simulink model "US53253_SimpleTorqueLimitingandGovernorControl"  (R2018b)
settings: Solver=ode45  StartTime=0.0  StopTime=10.0  RelTol=1e-3
undefined symbols (not defined in the file): DerivativeFilterGain_Gov, DerivativeFilterGain_Max, DerivativeFilterGain_Min, DerivativeFilterTimeConstant_Gov, DerivativeFilterTimeConstant_Max, DerivativeFilterTimeConstant_Min, DerivativeGainGovTable, DerivativeGainGovTable_X, DerivativeGainMaxTable, DerivativeGainMaxTable_X, DerivativeGainMinTable, DerivativeGainMinTable_X, DroopGovTable, DroopGovTable_X, DroopMaxTable, DroopMaxTable_X, DroopMinTable, DroopMinTable_X, FIZIT_GovSpeed, FIZIT_MaxSpeed, FIZIT_MinSpeed, FullThrottleSpeed_Gov, FullThrottleSpeed_Max, FullThrottleSpeed_Min, gov_maxspd, gov_minspd, GovTypeDefault, higpwr_C, higpwr_X, IntegralGainGovTable, IntegralGainGovTable_X, IntegralGainMinTable, IntegralGainMinTable_X, LIZIT_GovSpeed, LIZIT_MaxSpeed, LIZIT_MinSpeed, LowCoolantTempHysteresis, LowCoolantTempThreshold, lowpwr_C, lowpwr_X, LowSCRInletTempHysteresis, LowSCRInletTempThreshold, MinMaxTransitionHysteresis, nomfric_C, nomfric_X, nomfric_Y, NumberOfCylinders, ProportionalGainGovTable, ProportionalGainGovTable_X, ProportionalGainMaxTable, ProportionalGainMaxTable_X, ProportionalGainMinTable, ProportionalGainMinTable_X, SmkOp1_C, SmkOp1_X, SmkOp1_Y, ThrTqTbl_C, ThrTqTbl_X, ThrTqTbl_Y, TorqueToFuelConversionFactorInRangeTable_X ... (+8)
libraries: simulink x3, Filters x2
(part 1 of 2)
settings Model: Creator=ed50214  LastModifiedBy=dnyaneshwat2
settings DataIOCC: LimitDataPoints=on  SaveFormat=Array
settings OptimizationCC: BlockReduction=off  BooleanDataType=off  LifeSpan=inf
settings DebuggingCC: SaveWithParameterizedLinksMsg=none  UnderspecifiedInitializationDetection=Classic  MergeDetectMultiDrivingBlocksExec=none  SignalResolutionControl=TryResolveAllWithWarning  SFUnexpectedBacktrackingDiag=warning  SFNoUnconditionalDefaultTransitionDiag=warning  SFExecutionAtInitializationDiag=none
settings HardwareCC: ProdBitPerPointer=32  ProdBitPerSizeT=32  ProdBitPerPtrDiffT=32  ProdLargestAtomicFloat=None  ProdIntDivRoundTo=Undefined  ProdEndianess=Unspecified  ProdWordSize=32  ProdHWDeviceType=32-bit Generic  TargetUnknown=on
settings ModelReferenceCC: PropagateSignalLabelsOutOfModel=off
settings SFSimCC: SimUseLocalCustomCode=off
settings RTWCC: RTWUseLocalCustomCode=off
settings CodeAppCC: StateflowObjectComments=on
settings GRTTargetCC: TargetLangStandard=C89/C90 (ANSI)  GeneratePreprocessorConditionals=Disable all
settings ConfigComp: CovEnable=on  CovScope=ReferencedModels  RecordCoverage=on  CovMetricSettings=dw  CovHtmlReporting=on  CovSaveCumulativeToWorkspaceVar=on  CovSaveSingleToWorkspaceVar=on  CovExternalEMLEnable=off  CovSFcnEnable=off

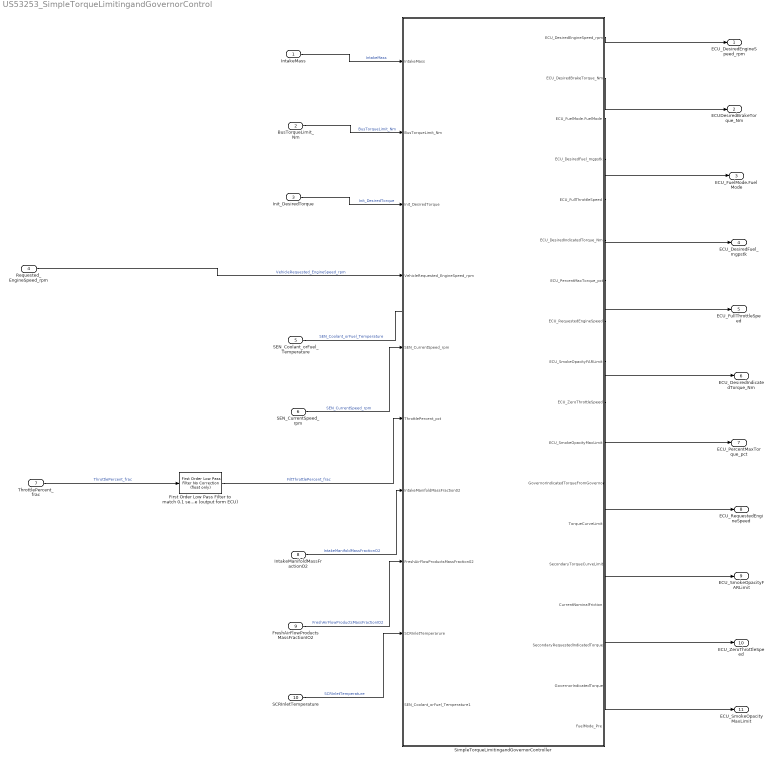
== system US53253_SimpleTorqueLimitingandGovernorControl ==
  IntakeMass : Inport
  BusTorqueLimit_Nm : Inport  Port=2
  Init_DesiredTorque : Inport  Port=3
  Requested_EngineSpeed_rpm : Inport  Port=4
  SEN_Coolant_orFuel_Temperature : Inport  Port=5
  SEN_CurrentSpeed_rpm : Inport  Port=6
  ThrottlePercent_frac : Inport  Port=7
  IntakeManifoldMassFractionO2 : Inport  Port=8
  FreshAirFlowProductsMassFractionIO2 : Inport  Port=9
  SCRInletTemperature : Inport  Port=10
  First Order Low Pass Filter to match 0.1 sec time constant in SiL from ThrottlePercent (input to ECU) to Throttle (output form ECU) : Filters/First Order Low Pass Filter No Correction (float only)  FilterGain=0.951229424500714  Filter_IC=0
      settings: SourceProductName=JDPS Filters
  SimpleTorqueLimitingandGovernorController : Subsystem  TreatAsAtomicUnit=on  mask(Engine control model){}
  ECU_DesiredEngineSpeed_rpm : Outport
  ECUDesiredBrakeTorque_Nm : Outport  Port=2
  ECU_FuelMode.FuelMode : Outport  Port=3
  ECU_DesiredFuel_mgpstk : Outport  Port=4
  ECU_FullThrottleSpeed : Outport  Port=5
  ECU_DesiredIndicatedTorque_Nm : Outport  Port=6
  ECU_PercentMaxTorque_pct : Outport  Port=7
  ECU_RequestedEngineSpeed : Outport  Port=8
  ECU_SmokeOpacityFARLimit : Outport  Port=9
  ECU_ZeroThrottleSpeed : Outport  Port=10
  ECU_SmokeOpacityMaxLimit : Outport  Port=11
  wires:
  IntakeMass/1 -> SimpleTorqueLimitingandGovernorController/1(IntakeMass)  "IntakeMass"
  BusTorqueLimit_Nm/1 -> SimpleTorqueLimitingandGovernorController/2(BusTorqueLimit_Nm)  "BusTorqueLimit_Nm"
  Init_DesiredTorque/1 -> SimpleTorqueLimitingandGovernorController/3(Init_DesiredTorque)  "Init_DesiredTorque"
  Requested_EngineSpeed_rpm/1 -> SimpleTorqueLimitingandGovernorController/4(VehicleRequested_EngineSpeed_rpm)  "VehicleRequested_EngineSpeed_rpm"
  SEN_Coolant_orFuel_Temperature/1 -> ?  "SEN_Coolant_orFuel_Temperature"
  SEN_CurrentSpeed_rpm/1 -> SimpleTorqueLimitingandGovernorController/5(SEN_CurrentSpeed_rpm)  "SEN_CurrentSpeed_rpm"
  IntakeManifoldMassFractionO2/1 -> SimpleTorqueLimitingandGovernorController/7(IntakeManifoldMassFraction02)  "IntakeManifoldMassFractionO2"
  FreshAirFlowProductsMassFractionIO2/1 -> SimpleTorqueLimitingandGovernorController/8(FreshAirFlowProductsMassFraction02)  "FreshAirFlowProductsMassFractionIO2"
  SCRInletTemperature/1 -> SimpleTorqueLimitingandGovernorController/9(SCRInletTemperarure)  "SCRInletTemperature"
  SimpleTorqueLimitingandGovernorController/1(ECU_DesiredEngineSpeed_rpm) -> ECU_DesiredEngineSpeed_rpm/1
  SimpleTorqueLimitingandGovernorController/2(ECU_DesiredBrakeTorque_Nm) -> ECUDesiredBrakeTorque_Nm/1
  SimpleTorqueLimitingandGovernorController/3(ECU_FuelMode.FuelMode) -> ECU_FuelMode.FuelMode/1
  SimpleTorqueLimitingandGovernorController/4(ECU_DesiredFuel_mgpstk) -> ECU_DesiredFuel_mgpstk/1
  SimpleTorqueLimitingandGovernorController/5(ECU_FullThrottleSpeed) -> ECU_FullThrottleSpeed/1
  SimpleTorqueLimitingandGovernorController/6(ECU_DesiredIndicatedTorque_Nm) -> ECU_DesiredIndicatedTorque_Nm/1
  SimpleTorqueLimitingandGovernorController/7(ECU_PercentMaxTorque_pct) -> ECU_PercentMaxTorque_pct/1
  SimpleTorqueLimitingandGovernorController/8(ECU_RequestedEngineSpeed) -> ECU_RequestedEngineSpeed/1
  SimpleTorqueLimitingandGovernorController/9(ECU_SmokeOpacityFARLimit) -> ECU_SmokeOpacityFARLimit/1
  SimpleTorqueLimitingandGovernorController/10(ECU_ZeroThrottleSpeed) -> ECU_ZeroThrottleSpeed/1
  SimpleTorqueLimitingandGovernorController/11(ECU_SmokeOpacityMaxLimit) -> ECU_SmokeOpacityMaxLimit/1
  ThrottlePercent_frac/1 -> First Order Low Pass Filter to match 0.1 sec time constant in SiL from ThrottlePercent (input to ECU) to Throttle (output form ECU)/1  "ThrottlePercent_frac"
  First Order Low Pass Filter to match 0.1 sec time constant in SiL from ThrottlePercent (input to ECU) to Throttle (output form ECU)/1 -> SimpleTorqueLimitingandGovernorController/6(ThrottlePercent_pct)  "FiltThrottlePercent_frac"

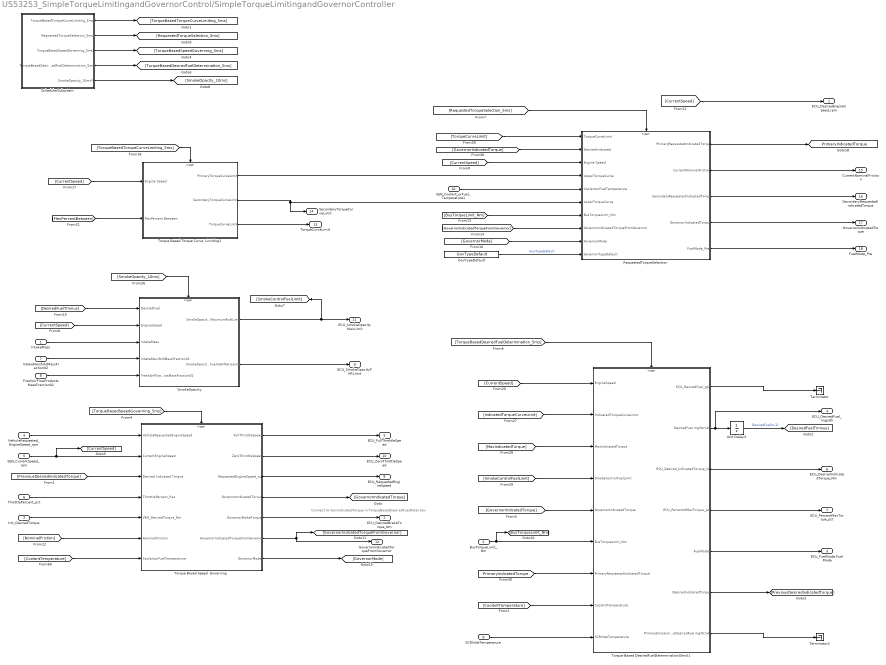
== system US53253_SimpleTorqueLimitingandGovernorControl/SimpleTorqueLimitingandGovernorController ==
  note: Connect to GovIndicatedTorque in TorqueBasedDesiredFuelDeter box
  IntakeMass : Inport
  BusTorqueLimit_Nm : Inport  Port=2
  Init_DesiredTorque : Inport  Port=3
  VehicleRequested_EngineSpeed_rpm : Inport  Port=4
  SEN_CurrentSpeed_rpm : Inport  Port=5
  ThrottlePercent_pct : Inport  Port=6
  IntakeManifoldMassFraction02 : Inport  Port=7
  FreshAirFlowProductsMassFraction02 : Inport  Port=8
  SCRInletTemperarure : Inport  Port=9
  SEN_Coolant_orFuel_Temperature1 : Inport  Port=10
  " Torque Based Speed  Governing" : Subsystem
  GovTypeDefault : Constant  Value=GovTypeDefault
  RequestedTorqueSelection : Subsystem
  SchedulerSubsytem : Stateflow chart  TreatAsAtomicUnit=on
  SmokeOpacity : Subsystem
  Terminator : Terminator
  Terminator2 : Terminator
  Torque Based DesiredFuelDetermination(5ms)1 : Subsystem
  Torque Based Torque Curve  Limiting1 : Subsystem
  Unit Delay3 : UnitDelay  InitialCondition=1000  SampleTime=-1
  ECU_DesiredEngineSpeed_rpm : Outport
  ECU_DesiredBrakeTorque_Nm : Outport  Port=2
  ECU_FuelMode.FuelMode : Outport  Port=3
  ECU_DesiredFuel_mgpstk : Outport  Port=4
  ECU_FullThrottleSpeed : Outport  Port=5
  ECU_DesiredIndicatedTorque_Nm : Outport  Port=6
  ECU_PercentMaxTorque_pct : Outport  Port=7
  ECU_RequestedEngineSpeed : Outport  Port=8
  ECU_SmokeOpacityFARLimit : Outport  Port=9
  ECU_ZeroThrottleSpeed : Outport  Port=10
  ECU_SmokeOpacityMaxLimit : Outport  Port=11
  GovernorIndicatedTorqueFromGovernor : Outport  Port=12
  TorqueCurveLimit : Outport  Port=13
  SecondaryTorqueCurveLimit : Outport  Port=14
  CurrentNominalFriction : Outport  Port=15
  SecondaryRequestedIndicatedTorque : Outport  Port=16
  GovernorIndicatedTorque : Outport  Port=17
  FuelMode_Pre : Outport  Port=18
  tag scope: PrimaryIndicatedTorque=global
  wires:
  [CurrentSpeed] -> ECU_DesiredEngineSpeed_rpm/1
  [SmokeOpacity_10ms] -> SmokeOpacity/Trigger
  [CurrentSpeed] -> SmokeOpacity/2(EngineSpeed)
  Unit Delay3/1 -> [DesiredFuelTminus]  "DesiredFuel(n-1)"
  [DesiredFuelTminus] -> SmokeOpacity/1(DesiredFuel)
  SmokeOpacity/2(SmokeOpacityFueltoAirRatioLimit) -> ECU_SmokeOpacityFARLimit/1
  Torque Based DesiredFuelDetermination(5ms)1/5(FuelMode) -> ECU_FuelMode.FuelMode/1
  Torque Based DesiredFuelDetermination(5ms)1/2(DesiredFuel mg/Stroke) -> ECU_DesiredFuel_mgpstk/1, Unit Delay3/1
  VehicleRequested_EngineSpeed_rpm/1 -> " Torque Based Speed  Governing"/1(VehicleRequestedEngineSpeed)
  SEN_CurrentSpeed_rpm/1 -> [CurrentSpeed], " Torque Based Speed  Governing"/2(CurrentEngineSpeed)
  Torque Based DesiredFuelDetermination(5ms)1/3(ECU_Desired_IndicatedTorque_Nm) -> ECU_DesiredIndicatedTorque_Nm/1
  Torque Based DesiredFuelDetermination(5ms)1/4(ECU_PercentofMaxTorque_pct) -> ECU_PercentMaxTorque_pct/1
  Torque Based DesiredFuelDetermination(5ms)1/7(PrimaryEmissionsMapDesiredFuel mg/Stroke) -> Terminator2/1
  [PreviousDesiredIndicatedTorque] -> " Torque Based Speed  Governing"/3(Desired Indicated Torque)
  " Torque Based Speed  Governing"/4(GovernorIndicatedTorque) -> [GovernorIndicatedTorque]
  [GovernorIndicatedTorque] -> Torque Based DesiredFuelDetermination(5ms)1/5(GovernorIndicatedTorque)
  Torque Based DesiredFuelDetermination(5ms)1/1(ECU_DesiredFuel_gps) -> Terminator/1
  [NominalFriction] -> " Torque Based Speed  Governing"/6(NominalFriction)
  Init_DesiredTorque/1 -> " Torque Based Speed  Governing"/5(VEH_DesiredTorque_Nm)
  BusTorqueLimit_Nm/1 -> [BusTorqueLimit_Nm], Torque Based DesiredFuelDetermination(5ms)1/6(BusTorqueLimit_Nm)
  IntakeMass/1 -> SmokeOpacity/3(IntakeMass)
  ThrottlePercent_pct/1 -> " Torque Based Speed  Governing"/4(ThrottlePercent_frac)
  " Torque Based Speed  Governing"/1(FullThrottleSpeed) -> ECU_FullThrottleSpeed/1
  " Torque Based Speed  Governing"/2(ZeroThrottleSpeed) -> ECU_ZeroThrottleSpeed/1
  " Torque Based Speed  Governing"/3(RequestedEngineSpeed_out) -> ECU_RequestedEngineSpeed/1
  [CurrentSpeed] -> Torque Based DesiredFuelDetermination(5ms)1/1(EngineSpeed)
  [PrimaryIndicatedTorque] -> Torque Based DesiredFuelDetermination(5ms)1/7(PrimaryRequestedIndicatedTorque)
  Torque Based DesiredFuelDetermination(5ms)1/6(DesiredIndicatedTorque) -> [PreviousDesiredIndicatedTorque]
  [IndicatedTorqueCurveLimit] -> Torque Based DesiredFuelDetermination(5ms)1/2(IndicatedTorqueCurveLimit)
  [SmokeControlFuelLimit] -> Torque Based DesiredFuelDetermination(5ms)1/4(SmokeControlFuelLimit)
  [MaxIndicatedTorque] -> Torque Based DesiredFuelDetermination(5ms)1/3(MaxIndicatedTorque)
  SmokeOpacity/1(SmokeOpacityMaximumFuelLimit) -> ECU_SmokeOpacityMaxLimit/1, [SmokeControlFuelLimit]
  [GovernorIndicatedTorque] -> RequestedTorqueSelection/2(DesiredInidcated)
  RequestedTorqueSelection/1(PrimaryRequestedIndicatedTorque) -> [PrimaryIndicatedTorque]
  [TorqueCurveLimit] -> RequestedTorqueSelection/1(TorqueCurveLimit)
  [CoolantTemperature] -> " Torque Based Speed  Governing"/7(CoolantorFuelTemperature)
  FreshAirFlowProductsMassFraction02/1 -> SmokeOpacity/5(FreshAirFlowProductsMassFraction02)
  IntakeManifoldMassFraction02/1 -> SmokeOpacity/4(IntakeManifoldMassFraction02)
  " Torque Based Speed  Governing"/5(GovernorBrakeTorque) -> ECU_DesiredBrakeTorque_Nm/1
  [CoolantTemperature] -> Torque Based DesiredFuelDetermination(5ms)1/8(CoolantTemperature)
  SCRInletTemperarure/1 -> Torque Based DesiredFuelDetermination(5ms)1/9(SCRInletTemperature)
  [TorqueBasedSpeedGoverning_5ms] -> " Torque Based Speed  Governing"/Trigger
  [TorqueBasedDesiredFuelDetermination_5ms] -> Torque Based DesiredFuelDetermination(5ms)1/Trigger
  [RequestedTorqueSelection_5ms] -> RequestedTorqueSelection/Trigger
  SchedulerSubsytem/1(TorqueBasedTorqueCurveLimiting_5ms()) -> [TorqueBasedTorqueCurveLimiting_5ms]
  SchedulerSubsytem/2(RequestedTorqueSelection_5ms()) -> [RequestedTorqueSelection_5ms]
  SchedulerSubsytem/3(TorqueBasedSpeedGoverning_5ms()) -> [TorqueBasedSpeedGoverning_5ms]
  SchedulerSubsytem/4(TorqueBasedDesiredFuelDetermination_5ms()) -> [TorqueBasedDesiredFuelDetermination_5ms]
  SchedulerSubsytem/5(SmokeOpacity_10ms()) -> [SmokeOpacity_10ms]
  [CurrentSpeed] -> RequestedTorqueSelection/3(Engine Speed)
  SEN_Coolant_orFuel_Temperature1/1 -> RequestedTorqueSelection/5(CoolantorFuelTemperature)
  [BusTorqueLimit_Nm] -> RequestedTorqueSelection/7(BusTorqueLimit_Nm)
  " Torque Based Speed  Governing"/6(GovernorIndicatedTorqueFromGovernor) -> GovernorIndicatedTorqueFromGovernor/1, [GovernorIndicatedTorqueFromGovernor]
  [GovernorIndicatedTorqueFromGovernor] -> RequestedTorqueSelection/8(GovernorIndicatedTorqueFromGovernor)
  [GovernorMode] -> RequestedTorqueSelection/9(GovernorMode)
  " Torque Based Speed  Governing"/7(GovernorMode) -> [GovernorMode]
  GovTypeDefault/1 -> RequestedTorqueSelection/10(GovernorTypeDefault)  "GovTypeDefault"
  Torque Based Torque Curve  Limiting1/2(SecondaryTorqueCurveLimit) -> RequestedTorqueSelection/6(LowerTorqueCurve), SecondaryTorqueCurveLimit/1
  Torque Based Torque Curve  Limiting1/3(TorqueCurveLimit) -> TorqueCurveLimit/1
  [TorqueBasedTorqueCurveLimiting_5ms] -> Torque Based Torque Curve  Limiting1/Trigger
  [FlexPercentBetween] -> Torque Based Torque Curve  Limiting1/2(FlexPercent Between)
  [CurrentSpeed] -> Torque Based Torque Curve  Limiting1/1(Engine Speed)
  Torque Based Torque Curve  Limiting1/1(PrimaryTorqueCurveLimit) -> RequestedTorqueSelection/4(UpperTorqueCurve)
  RequestedTorqueSelection/2(CurrentNominalFriction) -> CurrentNominalFriction/1
  RequestedTorqueSelection/3(SecondaryRequestedIndicatedTorque) -> SecondaryRequestedIndicatedTorque/1
  RequestedTorqueSelection/4(GovernorIndicatedTorque) -> GovernorIndicatedTorque/1
  RequestedTorqueSelection/5(FuelMode_Pre) -> FuelMode_Pre/1

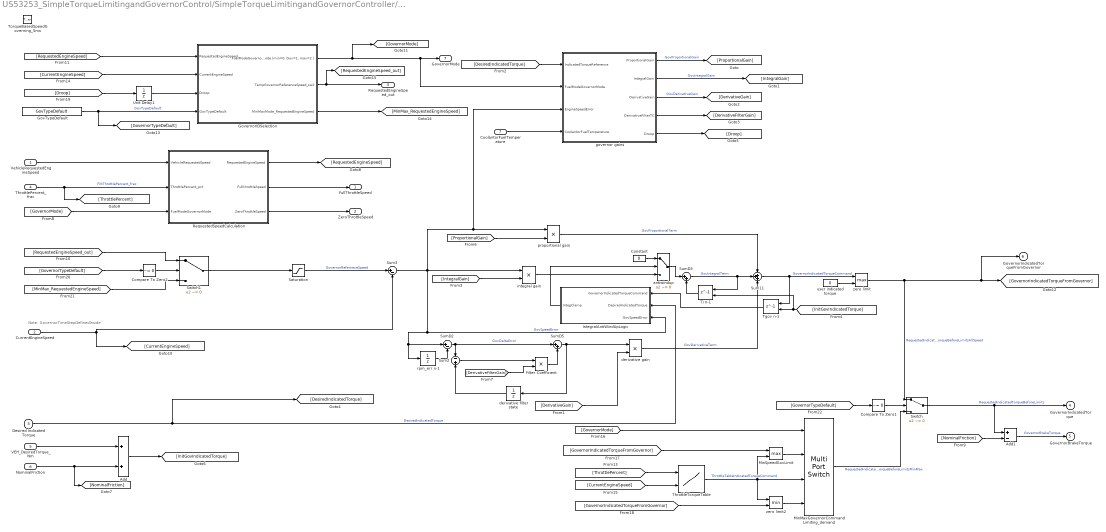
== system US53253_SimpleTorqueLimitingandGovernorControl/SimpleTorqueLimitingandGovernorController/ Torque Based Speed  Governing ==
  note: Note: GovernorTimeStepDefinedInside
  VehicleRequestedEngineSpeed : Inport
  CurrentEngineSpeed : Inport  Port=2
  Desired Indicated Torque : Inport  Port=3
  ThrottlePercent_frac : Inport  Port=4
  VEH_DesiredTorque_Nm : Inport  Port=5
  NominalFriction : Inport  Port=6
  CoolantorFuelTemperature : Inport  Port=7
  TorqueBasedSpeedGoverning_5ms : TriggerPort  TriggerType=function-call  VariantControl=(inherit)  PortDimensions=1
  Add : Sum
  Add1 : Sum  Inputs=+-
  Compare To Zero1 : simulink/Logic and Bit Operations/Compare To Zero  relop=~=  OutDataTypeStr=uint8
  Compare To Zero2 : simulink/Logic and Bit Operations/Compare To Zero  relop=~=  OutDataTypeStr=uint8
  Constant : Constant  Value=0
  Filter Coefficient : Product  Inputs=**  RndMeth=Zero
  GovTypeDefault : Constant  Value=GovTypeDefault
  GovernorIDSelection : Subsystem
  IntegralAntiWindUpLogic : Stateflow chart  TreatAsAtomicUnit=on
  MinMaxGovernorCommandLimiting_demand : MultiPortSwitch  DataPortOrder=Zero-based contiguous  zeroidx=on
  MinSpeedGovLimit : MinMax  Function=max  Inputs=2
  RequestedSpeedCalculation : Subsystem
  Saturation : Saturate  UpperLimit=gov_maxspd  LowerLimit=gov_minspd
      settings: AttributesFormatString=<lim: %<LowerLimit>/%<UpperLimit>>
  Sum11 : Sum  DisableCoverage=on  Inputs=+++
  Sum2 : Sum  Inputs=-+
  Sum3 : Sum  Inputs=|+-
  SumD2 : Sum  DisableCoverage=on  Inputs=|+-
  SumD3 : Sum  DisableCoverage=on  Inputs=|++
  SumD5 : Sum  DisableCoverage=on  Inputs=|++
  Switch : Switch  Criteria=u2 ~= 0
  Switch1 : Switch  Criteria=u2 ~= 0
  Tgov n-1 : Delay  DelayLength=1  InitialConditionSource=Input port
      settings: InputPortMap=u0,p4
  ThrottleTorqueTable : Lookup_n-D  BreakpointsForDimension1=ThrTqTbl_X  BreakpointsForDimension2=ThrTqTbl_Y  Table=ThrTqTbl_C  ExtrapMethod=Clip  UseLastTableValue=on  RndMeth=Simplest  InputSameDT=on
  Ti n-1 : Delay  DelayLength=1  InitialConditionSource=Input port
      settings: InputPortMap=u0,p4
  Unit Delay1 : UnitDelay  SampleTime=-1
  antiwindup : Switch  Criteria=u2 ~= 0
  derivative filter state : UnitDelay  SampleTime=-1
  derivative gain : Product  RndMeth=Zero
  governor gains : Subsystem
  integral gain : Product  RndMeth=Zero
  proportional gain : Product  RndMeth=Zero
  rpm_err n-1 : UnitDelay  SampleTime=-1
  user indicated torque : Constant  Value=0
  zero limit : MinMax  Function=max  Inputs=2
  zero limit2 : MinMax  Inputs=2
  FullThrottleSpeed : Outport
  ZeroThrottleSpeed : Outport  Port=2
  RequestedEngineSpeed_out : Outport  Port=3
  GovernorIndicatedTorque : Outport  Port=4  InitialOutput=0
  GovernorBrakeTorque : Outport  Port=5  InitialOutput=0
  GovernorIndicatedTorqueFromGovernor : Outport  Port=6  InitialOutput=0
  GovernorMode : Outport  Port=7
  wires:
  Desired Indicated Torque/1 -> [DesiredIndicatedTorque], IntegralAntiWindUpLogic/2(DesiredIndicatedTorque)  "DesiredIndicatedTorque"
  Tgov n-1/1 -> IntegralAntiWindUpLogic/1(GovernorIndicatedTorqueCommand)
  Ti n-1/1 -> SumD3/2
  Sum3/1 -> IntegralAntiWindUpLogic/3(GovSpeedError), SumD2/1, rpm_err n-1/1, integral gain/1, proportional gain/1, governor gains/3(EngineSpeedError)  "GovSpeedError"
  SumD3/1 -> Sum11/2, Ti n-1/1  "GovIntegralTerm"
  proportional gain/1 -> Sum11/1  "GovProportionalTerm"
  Sum11/1 -> zero limit/1, Tgov n-1/1  "GovernorIndicatedTorqueCommand"
  antiwindup/1 -> SumD3/1
  integral gain/1 -> antiwindup/3
  derivative gain/1 -> Sum11/3  "GovDerivativeTerm"
  Constant/1 -> antiwindup/1
  [ProportionalGain] -> proportional gain/2
  [IntegralGain] -> integral gain/2
  governor gains/1(ProportionalGain) -> [ProportionalGain]  "GovProportionalGain"
  CurrentEngineSpeed/1 -> [CurrentEngineSpeed], Sum3/2
  user indicated torque/1 -> zero limit/2
  [DerivativeGain] -> derivative gain/2
  governor gains/2(IntegralGain) -> [IntegralGain]  "GovIntegralGain"
  [DesiredIndicatedTorque] -> governor gains/1(IndicatedTorqueReference)
  governor gains/5(Droop) -> [Droop]
  governor gains/4(DerivativeFilterTC) -> [DerivativeFilterGain]
  governor gains/3(DerivativeGain) -> [DerivativeGain]  "GovDerivativeGain"
  SumD5/1 -> derivative filter state/1, derivative gain/1
  Sum2/1 -> Filter Coefficient/1
  [DerivativeFilterGain] -> Filter Coefficient/2
  SumD2/1 -> SumD5/1, Sum2/1  "GovDeltaError"
  rpm_err n-1/1 -> SumD2/2
  Saturation/1 -> Sum3/1  "GovernorReferneceSpeed"
  [InitGovIndicatedTorque] -> Tgov n-1/2, Ti n-1/2
  VehicleRequestedEngineSpeed/1 -> RequestedSpeedCalculation/1(VehicleRequestedSpeed)
  ThrottlePercent_frac/1 -> [ThrottlePercent], RequestedSpeedCalculation/2(ThrottlePercent_pct)  "FiltThrottlePercent_frac"
  [GovernorMode] -> RequestedSpeedCalculation/3(FuelModeGovernorMode)
  RequestedSpeedCalculation/1(RequestedEngineSpeed) -> [RequestedEngineSpeed]
  [RequestedEngineSpeed] -> GovernorIDSelection/1(RequestedEngineSpeed)
  RequestedSpeedCalculation/3(ZeroThrottleSpeed) -> ZeroThrottleSpeed/1
  RequestedSpeedCalculation/2(FullthrottleSpeed) -> FullThrottleSpeed/1
  CoolantorFuelTemperature/1 -> governor gains/4(CoolantorFuelTemperature)
  Compare To Zero1/1 -> Switch/2
  [ThrottlePercent] -> ThrottleTorqueTable/1
  [CurrentEngineSpeed] -> ThrottleTorqueTable/2
  [GovernorMode] -> MinMaxGovernorCommandLimiting_demand/1
  MinMaxGovernorCommandLimiting_demand/1 -> Switch/3  "RequestedIndicatedTorqueBeforeLimitsMinMax"
  ThrottleTorqueTable/1 -> MinSpeedGovLimit/2, zero limit2/1, MinMaxGovernorCommandLimiting_demand/3  "ThrottleTableIndicatedTorqueCommand"
  [GovernorIndicatedTorqueFromGovernor] -> MinSpeedGovLimit/1
  [GovernorIndicatedTorqueFromGovernor] -> zero limit2/2
  GovernorIDSelection/1("FuelModeGovernorMode (min=0, Gov=1, max=2 )") -> governor gains/2(FuelModeGovernorMode), GovernorMode/1, [GovernorMode]
  zero limit/1 -> GovernorIndicatedTorqueFromGovernor/1, [GovernorIndicatedTorqueFromGovernor], Switch/1  "RequestedIndicatedTorqueBeforeLimitsAllSpeed"
  Switch/1 -> Add1/1, GovernorIndicatedTorque/1  "RequestedIndicatedTorqueBeforeLimits"
  MinSpeedGovLimit/1 -> MinMaxGovernorCommandLimiting_demand/2
  zero limit2/1 -> MinMaxGovernorCommandLimiting_demand/4
  [CurrentEngineSpeed] -> GovernorIDSelection/2(CurrentEngineSpeed)
  [Droop] -> Unit Delay1/1
  Unit Delay1/1 -> GovernorIDSelection/3(Droop)
  GovernorIDSelection/3(MinMaxMode_RequestedEngineSpeed) -> [MinMax_RequestedEngineSpeed]
  [GovernorTypeDefault] -> Compare To Zero2/1
  Switch1/1 -> Saturation/1
  [RequestedEngineSpeed_out] -> Switch1/1
  Compare To Zero2/1 -> Switch1/2
  [MinMax_RequestedEngineSpeed] -> Switch1/3
  [GovernorTypeDefault] -> Compare To Zero1/1
  Add/1 -> [InitGovIndicatedTorque]
  VEH_DesiredTorque_Nm/1 -> Add/1
  NominalFriction/1 -> [NominalFriction], Add/2
  [NominalFriction] -> Add1/2
  Add1/1 -> GovernorBrakeTorque/1  "GovernorBrakeTorque"
  GovTypeDefault/1 -> [GovernorTypeDefault], GovernorIDSelection/4(GovTypeDefault)  "GovTypeDefault"
  Filter Coefficient/1 -> SumD5/2
  derivative filter state/1 -> Sum2/2
  GovernorIDSelection/2(TempGovernorReferenceSpeed_sw2) -> [RequestedEngineSpeed_out], RequestedEngineSpeed_out/1
  IntegralAntiWindUpLogic/1(IntegClamp) -> antiwindup/2

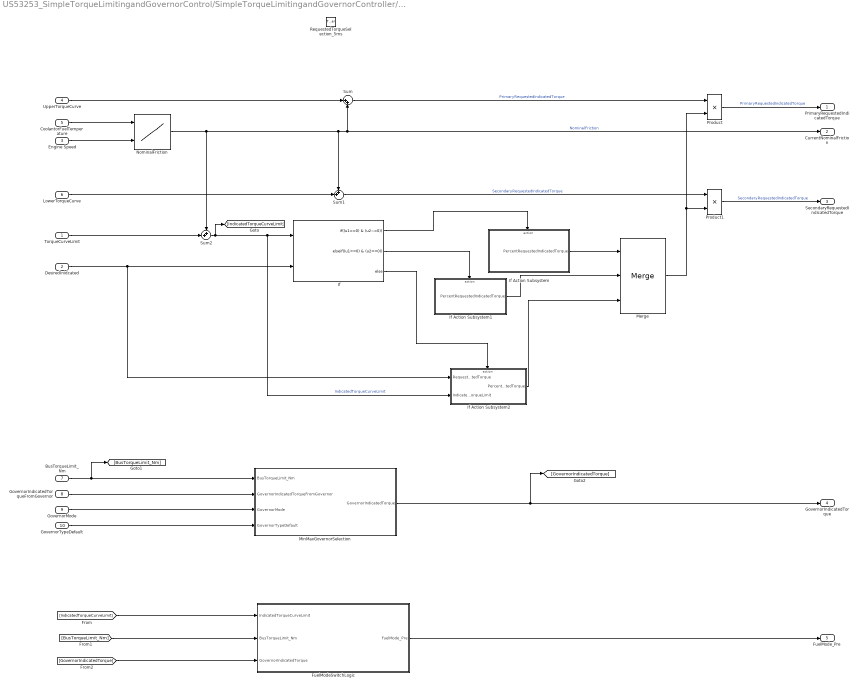
== system US53253_SimpleTorqueLimitingandGovernorControl/SimpleTorqueLimitingandGovernorController/RequestedTorqueSelection ==
  TorqueCurveLimit : Inport
  DesiredInidcated : Inport  Port=2
  Engine Speed : Inport  Port=3
  UpperTorqueCurve : Inport  Port=4
  CoolantorFuelTemperature : Inport  Port=5
  LowerTorqueCurve : Inport  Port=6
  BusTorqueLimit_Nm : Inport  Port=7
  GovernorIndicatedTorqueFromGovernor : Inport  Port=8
  GovernorMode : Inport  Port=9
  GovernorTypeDefault : Inport  Port=10
  RequestedTorqueSelection_5ms : TriggerPort  TriggerType=function-call  VariantControl=(inherit)  PortDimensions=1
  FuelModeSwitchLogic : Subsystem
  If : If  NumInputs=2  IfExpression=(u1==0) & (u2~=0)  ElseIfExpressions=(u1==0) & (u2==0)
  If Action Subsystem : Subsystem  TreatAsAtomicUnit=on
  If Action Subsystem1 : Subsystem  TreatAsAtomicUnit=on
  If Action Subsystem2 : Subsystem  TreatAsAtomicUnit=on
  Merge : Merge  Inputs=3
  MinMaxGovernorSelection : Subsystem
  NominalFriction : Lookup_n-D  BreakpointsForDimension1=nomfric_Y  BreakpointsForDimension2=nomfric_X  Table=nomfric_C  ExtrapMethod=Clip  UseLastTableValue=on  RndMeth=Simplest  InputSameDT=on
  Product : Product  RndMeth=Zero
  Product1 : Product  RndMeth=Zero
  Sum : Sum  Inputs=|++
  Sum1 : Sum  Inputs=++|
  Sum2 : Sum  Inputs=++|
  PrimaryRequestedIndicatedTorque : Outport
  CurrentNominalFriction : Outport  Port=2
  SecondaryRequestedIndicatedTorque : Outport  Port=3
  GovernorIndicatedTorque : Outport  Port=4
  FuelMode_Pre : Outport  Port=5
  wires:
  UpperTorqueCurve/1 -> Sum/1
  DesiredInidcated/1 -> If Action Subsystem2/1(RequestedIndicatedTorque), If/2
  TorqueCurveLimit/1 -> Sum2/2
  Sum/1 -> Product/1  "PrimaryRequestedIndicatedTorque"
  Product/1 -> PrimaryRequestedIndicatedTorque/1  "PrimaryRequestedIndicatedTorque"
  CoolantorFuelTemperature/1 -> NominalFriction/1
  Engine Speed/1 -> NominalFriction/2
  NominalFriction/1 -> CurrentNominalFriction/1, Sum/2, Sum1/1, Sum2/1  "NominalFriction"
  LowerTorqueCurve/1 -> Sum1/2
  If/1 -> If Action Subsystem/Action
  If Action Subsystem/1(PercentRequestedIndicatedTorque) -> Merge/1
  Product1/1 -> SecondaryRequestedIndicatedTorque/1  "SecondaryRequestedIndicatedTorque"
  Sum1/1 -> Product1/1  "SecondaryRequestedIndicatedTorque"
  If Action Subsystem1/1(PercentRequestedIndicatedTorque) -> Merge/2
  If Action Subsystem2/1(PercentRequestedIndicatedTorque) -> Merge/3
  If/3 -> If Action Subsystem2/Action
  If/2 -> If Action Subsystem1/Action
  Sum2/1 -> [IndicatedTorqueCurveLimit], If Action Subsystem2/2(IndicatedTorqueLimit), If/1  "IndicatedTorqueCurveLimit"
  Merge/1 -> Product/2, Product1/2
  [IndicatedTorqueCurveLimit] -> FuelModeSwitchLogic/1(IndicatedTorqueCurveLimit)
  [BusTorqueLimit_Nm] -> FuelModeSwitchLogic/2(BusTorqueLimit_Nm)
  [GovernorIndicatedTorque] -> FuelModeSwitchLogic/3(GovernorIndicatedTorque)
  FuelModeSwitchLogic/1(FuelMode_Pre) -> FuelMode_Pre/1
  BusTorqueLimit_Nm/1 -> [BusTorqueLimit_Nm], MinMaxGovernorSelection/1(BusTorqueLimit_Nm)
  GovernorIndicatedTorqueFromGovernor/1 -> MinMaxGovernorSelection/2(GovernorIndicatedTorqueFromGovernor)
  GovernorMode/1 -> MinMaxGovernorSelection/3(GovernorMode)
  GovernorTypeDefault/1 -> MinMaxGovernorSelection/4(GovernorTypeDefault)
  MinMaxGovernorSelection/1(GovernorIndicatedTorque) -> [GovernorIndicatedTorque], GovernorIndicatedTorque/1

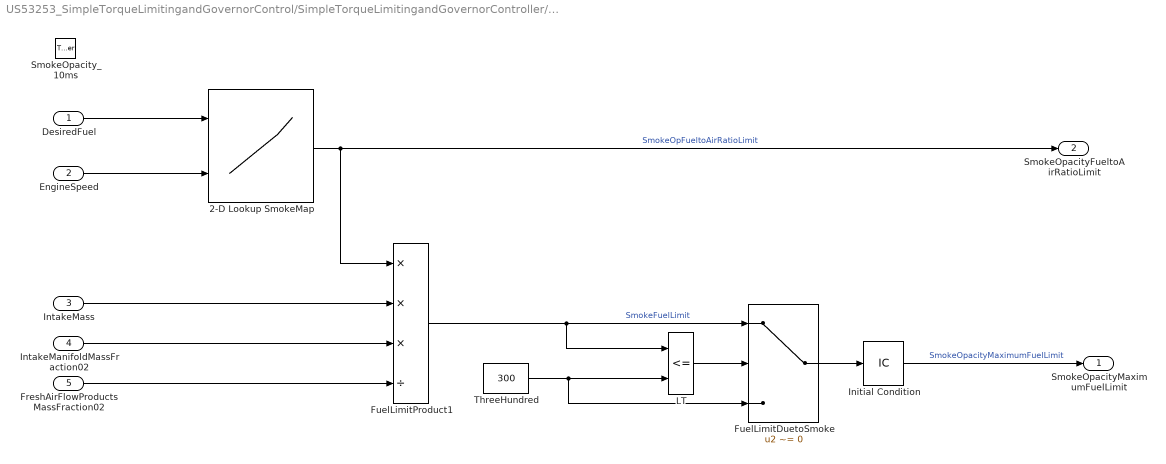
== system US53253_SimpleTorqueLimitingandGovernorControl/SimpleTorqueLimitingandGovernorController/SmokeOpacity ==
  DesiredFuel : Inport
  EngineSpeed : Inport  Port=2
  IntakeMass : Inport  Port=3
  IntakeManifoldMassFraction02 : Inport  Port=4
  FreshAirFlowProductsMassFraction02 : Inport  Port=5
  SmokeOpacity_10ms : TriggerPort  TriggerType=function-call  VariantControl=(inherit)  PortDimensions=1
  2-D Lookup SmokeMap : Lookup_n-D  BreakpointsForDimension1=SmkOp1_Y  BreakpointsForDimension2=SmkOp1_X  Table=SmkOp1_C  ExtrapMethod=Clip  UseLastTableValue=on  RndMeth=Simplest  InputSameDT=on
  FuelLimitDuetoSmoke : Switch  Criteria=u2 ~= 0
  FuelLimitProduct1 : Product  Inputs=***/  SaturateOnIntegerOverflow=on
  Initial Condition : InitialCondition  Value=500
  LT : RelationalOperator  Operator=<=  OutDataTypeStr=boolean  RndMeth=Nearest
  ThreeHundred : Constant  Value=300
  SmokeOpacityMaximumFuelLimit : Outport
  SmokeOpacityFueltoAirRatioLimit : Outport  Port=2
  wires:
  DesiredFuel/1 -> 2-D Lookup SmokeMap/1
  EngineSpeed/1 -> 2-D Lookup SmokeMap/2
  2-D Lookup SmokeMap/1 -> SmokeOpacityFueltoAirRatioLimit/1, FuelLimitProduct1/1  "SmokeOpFueltoAirRatioLimit"
  FuelLimitDuetoSmoke/1 -> Initial Condition/1
  LT/1 -> FuelLimitDuetoSmoke/2
  ThreeHundred/1 -> LT/2, FuelLimitDuetoSmoke/3
  FuelLimitProduct1/1 -> LT/1, FuelLimitDuetoSmoke/1  "SmokeFuelLimit"
  IntakeMass/1 -> FuelLimitProduct1/2
  IntakeManifoldMassFraction02/1 -> FuelLimitProduct1/3
  FreshAirFlowProductsMassFraction02/1 -> FuelLimitProduct1/4
  Initial Condition/1 -> SmokeOpacityMaximumFuelLimit/1  "SmokeOpacityMaximumFuelLimit"

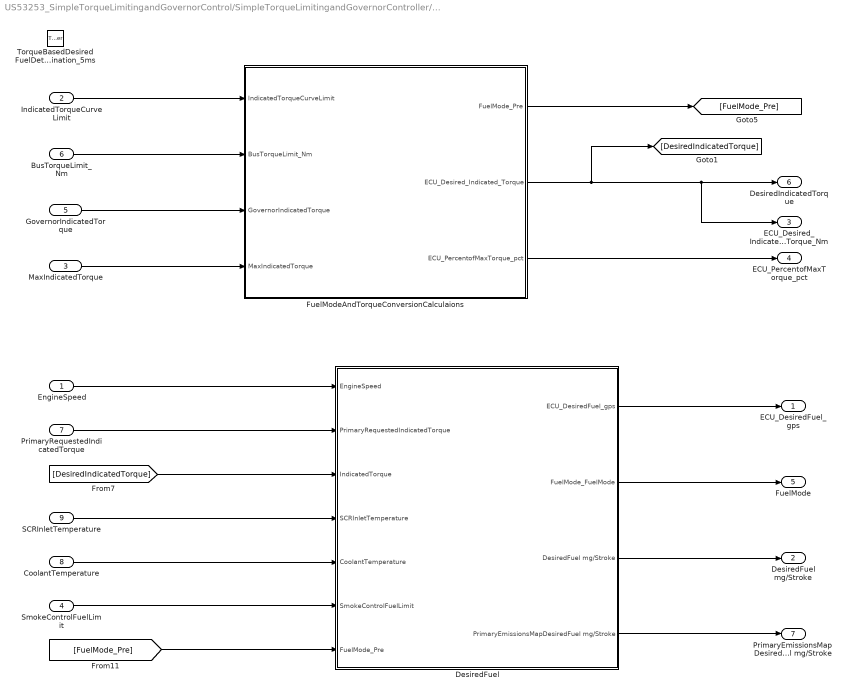
== system US53253_SimpleTorqueLimitingandGovernorControl/SimpleTorqueLimitingandGovernorController/Torque Based DesiredFuelDetermination(5ms)1 ==
  EngineSpeed : Inport
  IndicatedTorqueCurveLimit : Inport  Port=2
  MaxIndicatedTorque : Inport  Port=3
  SmokeControlFuelLimit : Inport  Port=4
  GovernorIndicatedTorque : Inport  Port=5
  BusTorqueLimit_Nm : Inport  Port=6
  PrimaryRequestedIndicatedTorque : Inport  Port=7
  CoolantTemperature : Inport  Port=8
  SCRInletTemperature : Inport  Port=9
  TorqueBasedDesiredFuelDetermination_5ms : TriggerPort  TriggerType=function-call  VariantControl=(inherit)  PortDimensions=1
  DesiredFuel : Subsystem
  FuelModeAndTorqueConversionCalculaions : Subsystem
  ECU_DesiredFuel_gps : Outport
  DesiredFuel mg/Stroke : Outport  Port=2
  ECU_Desired_IndicatedTorque_Nm : Outport  Port=3
  ECU_PercentofMaxTorque_pct : Outport  Port=4
  FuelMode : Outport  Port=5
  DesiredIndicatedTorque : Outport  Port=6
  PrimaryEmissionsMapDesiredFuel mg/Stroke : Outport  Port=7
  wires:
  EngineSpeed/1 -> DesiredFuel/1(EngineSpeed)
  [DesiredIndicatedTorque] -> DesiredFuel/3(IndicatedTorque)
  PrimaryRequestedIndicatedTorque/1 -> DesiredFuel/2(PrimaryRequestedIndicatedTorque)
  SCRInletTemperature/1 -> DesiredFuel/4(SCRInletTemperature)
  CoolantTemperature/1 -> DesiredFuel/5(CoolantTemperature)
  FuelModeAndTorqueConversionCalculaions/2(ECU_Desired_Indicated_Torque) -> [DesiredIndicatedTorque], ECU_Desired_IndicatedTorque_Nm/1, DesiredIndicatedTorque/1
  IndicatedTorqueCurveLimit/1 -> FuelModeAndTorqueConversionCalculaions/1(IndicatedTorqueCurveLimit)
  BusTorqueLimit_Nm/1 -> FuelModeAndTorqueConversionCalculaions/2(BusTorqueLimit_Nm)
  GovernorIndicatedTorque/1 -> FuelModeAndTorqueConversionCalculaions/3(GovernorIndicatedTorque)
  MaxIndicatedTorque/1 -> FuelModeAndTorqueConversionCalculaions/4(MaxIndicatedTorque)
  FuelModeAndTorqueConversionCalculaions/1(FuelMode_Pre) -> [FuelMode_Pre]
  FuelModeAndTorqueConversionCalculaions/3(ECU_PercentofMaxTorque_pct) -> ECU_PercentofMaxTorque_pct/1
  DesiredFuel/1(ECU_DesiredFuel_gps) -> ECU_DesiredFuel_gps/1
  DesiredFuel/2(FuelMode_FuelMode) -> FuelMode/1
  DesiredFuel/3(DesiredFuel mg/Stroke) -> DesiredFuel mg/Stroke/1
  DesiredFuel/4(PrimaryEmissionsMapDesiredFuel mg/Stroke) -> PrimaryEmissionsMapDesiredFuel mg/Stroke/1
  SmokeControlFuelLimit/1 -> DesiredFuel/6(SmokeControlFuelLimit)
  [FuelMode_Pre] -> DesiredFuel/7(FuelMode_Pre)

== system US53253_SimpleTorqueLimitingandGovernorControl/SimpleTorqueLimitingandGovernorController/Torque Based Torque Curve  Limiting1 ==
  Engine Speed : Inport
  FlexPercent Between : Inport  Port=2
  TorqueBasedTorqueCurveLimiting_5ms : TriggerPort  TriggerType=function-call  VariantControl=(inherit)  PortDimensions=1
  Lower Curve : Lookup  InputValues=lowpwr_X  Table=lowpwr_C  LookUpMeth=Interpolation-Use End Values
  Product : Product
  Sum1 : Sum  Inputs=|+-
  Sum2 : Sum  Inputs=|++
  Upper Curve : Lookup  InputValues=higpwr_X  Table=higpwr_C  LookUpMeth=Interpolation-Use End Values
  PrimaryTorqueCurveLimit : Outport
  SecondaryTorqueCurveLimit : Outport  Port=2
  TorqueCurveLimit : Outport  Port=3
  wires:
  Engine Speed/1 -> Upper Curve/1, Lower Curve/1
  Upper Curve/1 -> PrimaryTorqueCurveLimit/1, Sum1/1  "UpperTorqueCurve"
  Lower Curve/1 -> SecondaryTorqueCurveLimit/1, Sum2/2, Sum1/2  "LowerTorqueCurve"
  Sum1/1 -> Product/2
  FlexPercent Between/1 -> Product/1
  Product/1 -> Sum2/1
  Sum2/1 -> TorqueCurveLimit/1

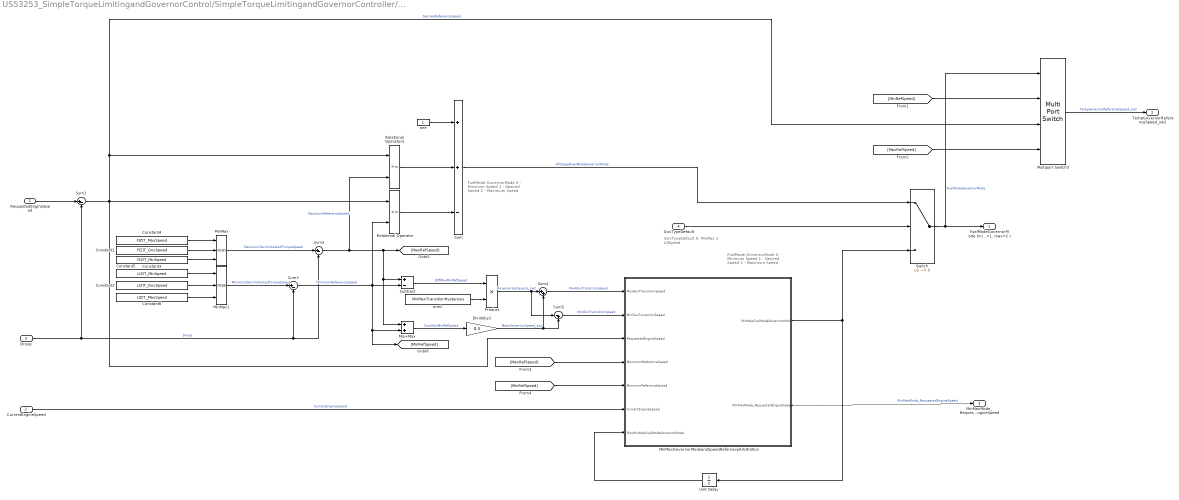
== system US53253_SimpleTorqueLimitingandGovernorControl/SimpleTorqueLimitingandGovernorController/ Torque Based Speed  Governing/GovernorIDSelection ==
  note: FuelMode.GovernorMode
      | 0 - Minimum Speed
      | 1 - Desired Speed
      | 2 - Maximum Speed
  note: GovTypeDefault
      | 0: MinMax
      | 1: AllSpeed
  note: FuelMode.GovernorMode
      | 0 - Minimum Speed
      | 1 - Desired Speed
      | 2 - Maximum Speed
  RequestedEngineSpeed : Inport
  CurrentEngineSpeed : Inport  Port=2
  Droop : Inport  Port=3
  GovTypeDefault : Inport  Port=4
  Constant1 : Constant  Value=FIZIT_GovSpeed
  Constant2 : Constant  Value=LIZIT_GovSpeed
  Constant3 : Constant  Value=FIZIT_MinSpeed
  Constant4 : Constant  Value=FIZIT_MaxSpeed
  Constant5 : Constant  Value=LIZIT_MinSpeed
  Constant6 : Constant  Value=LIZIT_MaxSpeed
  Divideby2 : Gain  Gain=0.5
  MInMaxGovernorModeandSpeedReferneceArbitration : Stateflow chart  TreatAsAtomicUnit=on
  Min+Max : Sum
  MinMax : MinMax  Inputs=3
  MinMax1 : MinMax  Function=max  Inputs=3
  Multiport Switch3 : MultiPortSwitch  DataPortOrder=Zero-based contiguous  zeroidx=on
  Product : Product  RndMeth=Zero
  Relational Operator : RelationalOperator  Operator=<=  RndMeth=Nearest
  Relational Operator5 : RelationalOperator  RndMeth=Nearest
  Subtract : Sum  Inputs=+-
  Sum : Sum  Inputs=++-
  Sum1 : Sum  Inputs=|+-
  Sum2 : Sum  Inputs=|+-
  Sum3 : Sum  Inputs=|+-
  Sum4 : Sum  Inputs=|++
  Sum5 : Sum  Inputs=|-+
  Switch : Switch  Criteria=u2 ~= 0
  Unit Delay : UnitDelay  SampleTime=-1
  one : Constant
  one2 : Constant  Description=Hysteresis  Value=MinMaxTransitionHysteresis
  "FuelModeGovernorMode (min=0, Gov=1, max=2 )" : Outport
  TempGovernorReferenceSpeed_sw2 : Outport  Port=2
  MinMaxMode_RequestedEngineSpeed : Outport  Port=3
  wires:
  one/1 -> Sum/1
  GovTypeDefault/1 -> Switch/2
  Switch/1 -> Multiport Switch3/1, "FuelModeGovernorMode (min=0, Gov=1, max=2 )"/1  "FuelModeGovernorMode"
  Sum/1 -> Switch/1  "AllSpeedFuelModeGovernorMode"
  Droop/1 -> Sum1/2, Sum2/2, Sum3/2  "Droop"
  Sum2/1 -> Subtract/1, Min+Max/1, [MaxRefSpeed], Relational Operator5/2  "MaximumReferenceSpeed"
  Sum3/1 -> Subtract/2, Min+Max/2, [MinRefSpeed], Relational Operator/2  "MinimumReferenceSpeed"
  Subtract/1 -> Product/1  "DiffMaxMinRefSpeed"
  one2/1 -> Product/2
  Min+Max/1 -> Divideby2/1  "SumMaxMinRefSpeed"
  Product/1 -> Sum4/1, Sum5/1  "GovernorHysteresis_sw2"
  Divideby2/1 -> Sum5/2, Sum4/2  "MeanGovernorSpeed_sw2"
  Sum4/1 -> MInMaxGovernorModeandSpeedReferneceArbitration/1(MaxGovTransitionSpeed)  "MaxGovTransitionSpeed"
  Sum5/1 -> MInMaxGovernorModeandSpeedReferneceArbitration/2(MinGovTransitionSpeed)  "MinGovTransitionSpeed"
  MInMaxGovernorModeandSpeedReferneceArbitration/2(MinMaxMode_RequestedEngineSpeed) -> MinMaxMode_RequestedEngineSpeed/1  "MinMaxMode_RequestedEngineSpeed"
  [MinRefSpeed] -> MInMaxGovernorModeandSpeedReferneceArbitration/5(MinimumReferenceSpeed)
  [MaxRefSpeed] -> MInMaxGovernorModeandSpeedReferneceArbitration/4(MaximumReferenceSpeed)
  Sum1/1 -> MInMaxGovernorModeandSpeedReferneceArbitration/3(RequestedEngineSpeed), Multiport Switch3/3, Relational Operator5/1, Relational Operator/1  "DesiredReferenceSpeed"
  Constant3/1 -> MinMax/3
  Constant1/1 -> MinMax/2
  Constant4/1 -> MinMax/1
  Constant5/1 -> MinMax1/1
  Constant2/1 -> MinMax1/2
  Constant6/1 -> MinMax1/3
  Relational Operator/1 -> Sum/3
  MinMax/1 -> Sum2/1  "MaximumZeroIndicatedTorqueSpeed"
  Relational Operator5/1 -> Sum/2
  MinMax1/1 -> Sum3/1  "MinimumZeroIndicatedTorqueSpeed"
  Multiport Switch3/1 -> TempGovernorReferenceSpeed_sw2/1  "TempGovernorReferenceSpeed_sw2"
  [MinRefSpeed] -> Multiport Switch3/2
  [MaxRefSpeed] -> Multiport Switch3/4
  MInMaxGovernorModeandSpeedReferneceArbitration/1(MinMaxFuelModeGovernorMode) -> Switch/3, Unit Delay/1
  CurrentEngineSpeed/1 -> MInMaxGovernorModeandSpeedReferneceArbitration/6(CurrentEngineSpeed)  "CurrentEngineSpeed"
  Unit Delay/1 -> MInMaxGovernorModeandSpeedReferneceArbitration/7(PrevMinMaxFuelModeGovernorMode)
  RequestedEngineSpeed/1 -> Sum1/1

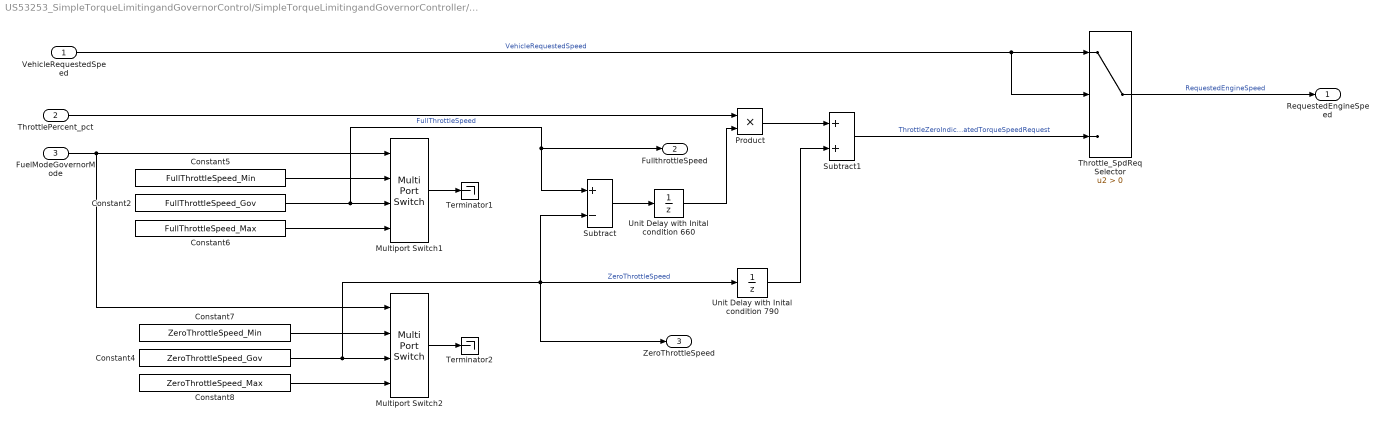
== system US53253_SimpleTorqueLimitingandGovernorControl/SimpleTorqueLimitingandGovernorController/ Torque Based Speed  Governing/RequestedSpeedCalculation ==
  VehicleRequestedSpeed : Inport
  ThrottlePercent_pct : Inport  Port=2
  FuelModeGovernorMode : Inport  Port=3
  Constant2 : Constant  Value=FullThrottleSpeed_Gov
  Constant4 : Constant  Value=ZeroThrottleSpeed_Gov
  Constant5 : Constant  Value=FullThrottleSpeed_Min
  Constant6 : Constant  Value=FullThrottleSpeed_Max
  Constant7 : Constant  Value=ZeroThrottleSpeed_Min
  Constant8 : Constant  Value=ZeroThrottleSpeed_Max
  Multiport Switch1 : MultiPortSwitch  DataPortOrder=Zero-based contiguous  zeroidx=on
  Multiport Switch2 : MultiPortSwitch  DataPortOrder=Zero-based contiguous  zeroidx=on
  Product : Product  RndMeth=Zero
  Subtract : Sum  Inputs=+-
  Subtract1 : Sum
  Terminator1 : Terminator
  Terminator2 : Terminator
  Throttle_SpdReq Selector : Switch  Criteria=u2 > Threshold
  Unit Delay with Inital condition 660 : UnitDelay  InitialCondition=660  SampleTime=-1
  Unit Delay with Inital condition 790 : UnitDelay  InitialCondition=790  SampleTime=-1
  RequestedEngineSpeed : Outport
  FullthrottleSpeed : Outport  Port=2
  ZeroThrottleSpeed : Outport  Port=3
  wires:
  VehicleRequestedSpeed/1 -> Throttle_SpdReq Selector/2, Throttle_SpdReq Selector/1  "VehicleRequestedSpeed"
  ThrottlePercent_pct/1 -> Product/1
  Constant2/1 -> Multiport Switch1/3, Subtract/1, FullthrottleSpeed/1  "FullThrottleSpeed"
  Constant4/1 -> ZeroThrottleSpeed/1, Unit Delay with Inital condition 790/1, Subtract/2, Multiport Switch2/3  "ZeroThrottleSpeed"
  Product/1 -> Subtract1/1
  Subtract1/1 -> Throttle_SpdReq Selector/3  "ThrottleZeroIndicatedTorqueSpeedRequest"
  Throttle_SpdReq Selector/1 -> RequestedEngineSpeed/1  "RequestedEngineSpeed"
  Unit Delay with Inital condition 790/1 -> Subtract1/2
  Subtract/1 -> Unit Delay with Inital condition 660/1
  Unit Delay with Inital condition 660/1 -> Product/2
  Constant5/1 -> Multiport Switch1/2
  Constant7/1 -> Multiport Switch2/2
  Constant8/1 -> Multiport Switch2/4
  FuelModeGovernorMode/1 -> Multiport Switch1/1, Multiport Switch2/1
  Constant6/1 -> Multiport Switch1/4
  Multiport Switch1/1 -> Terminator1/1
  Multiport Switch2/1 -> Terminator2/1

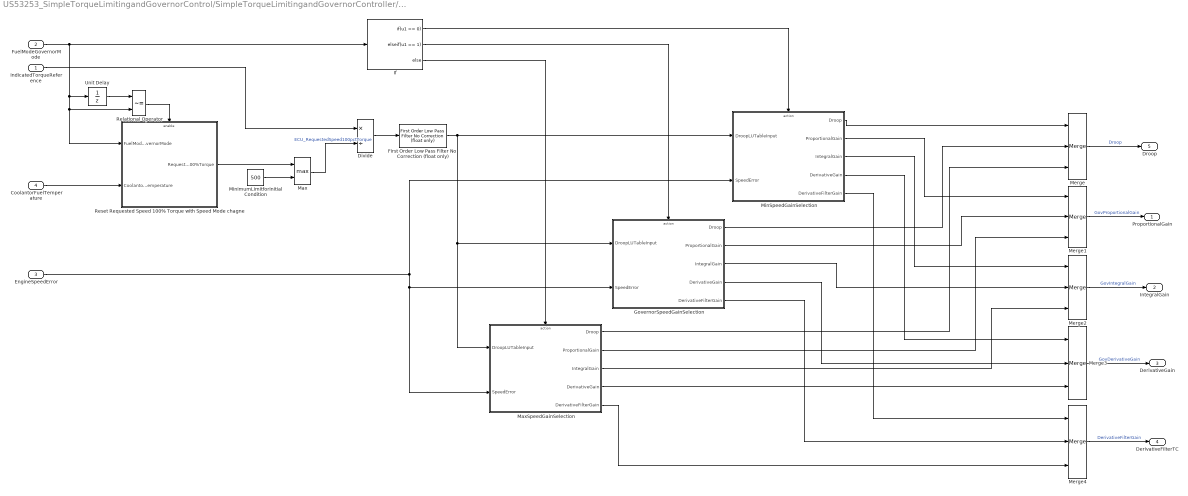
== system US53253_SimpleTorqueLimitingandGovernorControl/SimpleTorqueLimitingandGovernorController/ Torque Based Speed  Governing/governor gains ==
  IndicatedTorqueReference : Inport
  FuelModeGovernorMode : Inport  Port=2
  EngineSpeedError : Inport  Port=3
  CoolantorFuelTemperature : Inport  Port=4
  Divide : Product  Inputs=*/
  First Order Low Pass Filter No Correction (float only) : Filters/First Order Low Pass Filter No Correction (float only)  FilterGain=RequestedIndicatedTorqueFilterGain  Filter_IC=0
      settings: SourceProductName=JDPS Filters
  GovernorSpeedGainSelection : Subsystem  TreatAsAtomicUnit=on
  If : If  IfExpression=u1 == 0  ElseIfExpressions=u1 == 1
  Max : MinMax  Function=max  Inputs=2  ZeroCross=off
  MaxSpeedGainSelection : Subsystem  TreatAsAtomicUnit=on
  Merge{,1..4} (5 alike) : Merge  Inputs=3
  MinSpeedGainSelection : Subsystem  TreatAsAtomicUnit=on
  MinimumLimitforInitialCondition : Constant  Value=500
  Relational Operator : RelationalOperator  Operator=~=  OutDataTypeStr=boolean  RndMeth=Nearest
  Reset Requested Speed 100% Torque with Speed Mode chagne : Subsystem  TreatAsAtomicUnit=on
  Unit Delay : UnitDelay  InitialCondition=-1  SampleTime=-1
  ProportionalGain : Outport
  IntegralGain : Outport  Port=2
  DerivativeGain : Outport  Port=3
  DerivativeFilterTC : Outport  Port=4
  Droop : Outport  Port=5
  wires:
  FuelModeGovernorMode/1 -> If/1, Unit Delay/1, Reset Requested Speed 100% Torque with Speed Mode chagne/1(FuelModeGovernorMode), Relational Operator/2
  Divide/1 -> First Order Low Pass Filter No Correction (float only)/1
  IndicatedTorqueReference/1 -> Divide/1
  Unit Delay/1 -> Relational Operator/1
  Relational Operator/1 -> Reset Requested Speed 100% Torque with Speed Mode chagne/Enable
  MinimumLimitforInitialCondition/1 -> Max/2
  Reset Requested Speed 100% Torque with Speed Mode chagne/1(RequestedSpeed100%Torque) -> Max/1
  Max/1 -> Divide/2  "ECU_RequestedSpeed100pctTorque"
  CoolantorFuelTemperature/1 -> Reset Requested Speed 100% Torque with Speed Mode chagne/2(CoolantorFuelTemperature)
  If/1 -> MinSpeedGainSelection/Action
  If/2 -> GovernorSpeedGainSelection/Action
  If/3 -> MaxSpeedGainSelection/Action
  EngineSpeedError/1 -> MaxSpeedGainSelection/2(SpeedError), GovernorSpeedGainSelection/2(SpeedError), MinSpeedGainSelection/2(SpeedError)
  First Order Low Pass Filter No Correction (float only)/1 -> GovernorSpeedGainSelection/1(DroopLUTableInput), MaxSpeedGainSelection/1(DroopLUTableInput), MinSpeedGainSelection/1(DroopLUTableInput)
  Merge/1 -> Droop/1  "Droop"
  Merge1/1 -> ProportionalGain/1  "GovProportionalGain"
  Merge2/1 -> IntegralGain/1  "GovIntegralGain"
  Merge3/1 -> DerivativeGain/1  "GovDerivativeGain"
  MinSpeedGainSelection/1(Droop) -> Merge/1
  MaxSpeedGainSelection/1(Droop) -> Merge/3
  GovernorSpeedGainSelection/1(Droop) -> Merge/2
  MinSpeedGainSelection/2(ProportionalGain) -> Merge1/1
  GovernorSpeedGainSelection/2(ProportionalGain) -> Merge1/2
  MaxSpeedGainSelection/2(ProportionalGain) -> Merge1/3
  MinSpeedGainSelection/3(IntegralGain) -> Merge2/1
  GovernorSpeedGainSelection/3(IntegralGain) -> Merge2/2
  MaxSpeedGainSelection/3(IntegralGain) -> Merge2/3
  GovernorSpeedGainSelection/4(DerivativeGain) -> Merge3/2
  MinSpeedGainSelection/4(DerivativeGain) -> Merge3/1
  MaxSpeedGainSelection/4(DerivativeGain) -> Merge3/3
  MinSpeedGainSelection/5(DerivativeFilterGain) -> Merge4/1
  GovernorSpeedGainSelection/5(DerivativeFilterGain) -> Merge4/2
  MaxSpeedGainSelection/5(DerivativeFilterGain) -> Merge4/3
  Merge4/1 -> DerivativeFilterTC/1  "DerivativeFilterGain"

== system US53253_SimpleTorqueLimitingandGovernorControl/SimpleTorqueLimitingandGovernorController/RequestedTorqueSelection/FuelModeSwitchLogic ==
  IndicatedTorqueCurveLimit : Inport
  BusTorqueLimit_Nm : Inport  Port=2
  GovernorIndicatedTorque : Inport  Port=3
  Governor : Constant  Value=2
  GovernorLimited : Constant  Value=4
  Relational Operator : RelationalOperator  Operator=<=  OutDataTypeStr=boolean  RndMeth=Nearest
  Relational Operator1 : RelationalOperator  Operator=<=  OutDataTypeStr=boolean  RndMeth=Nearest
  Switch1 : Switch  Criteria=u2 ~= 0
  Switch2 : Switch  Criteria=u2 ~= 0
  TorqueLimited : Constant  Value=8
  curve limit2 : MinMax  Inputs=2
  FuelMode_Pre : Outport
  wires:
  Governor/1 -> Switch2/3
  Relational Operator/1 -> Switch1/2
  Relational Operator1/1 -> Switch2/2
  BusTorqueLimit_Nm/1 -> curve limit2/2, Relational Operator/2
  GovernorLimited/1 -> Switch1/3
  Switch1/1 -> Switch2/1
  TorqueLimited/1 -> Switch1/1
  curve limit2/1 -> Relational Operator1/1  "ECU_Torque_Curve_Limit"
  Switch2/1 -> FuelMode_Pre/1  "FuelMode_Pre"
  IndicatedTorqueCurveLimit/1 -> curve limit2/1, Relational Operator/1
  GovernorIndicatedTorque/1 -> Relational Operator1/2

== system US53253_SimpleTorqueLimitingandGovernorControl/SimpleTorqueLimitingandGovernorController/RequestedTorqueSelection/If Action Subsystem ==
  Action Port : ActionPort  ActionType=then
  Constant : Constant  Value=1.0
  PercentRequestedIndicatedTorque : Outport
  wires:
  Constant/1 -> PercentRequestedIndicatedTorque/1

== system US53253_SimpleTorqueLimitingandGovernorControl/SimpleTorqueLimitingandGovernorController/RequestedTorqueSelection/If Action Subsystem1 ==
  Action Port : ActionPort  ActionType=elseif
  Constant : Constant  Value=0.0
  PercentRequestedIndicatedTorque : Outport
  wires:
  Constant/1 -> PercentRequestedIndicatedTorque/1

== system US53253_SimpleTorqueLimitingandGovernorControl/SimpleTorqueLimitingandGovernorController/RequestedTorqueSelection/If Action Subsystem2 ==
  RequestedIndicatedTorque : Inport
  IndicatedTorqueLimit : Inport  Port=2
  Action Port : ActionPort  ActionType=else
  Divide : Product  Inputs=*/
  PercentRequestedIndicatedTorque : Outport
  wires:
  RequestedIndicatedTorque/1 -> Divide/1
  IndicatedTorqueLimit/1 -> Divide/2
  Divide/1 -> PercentRequestedIndicatedTorque/1  "PercentRequestedIndicatedTorque"

== system US53253_SimpleTorqueLimitingandGovernorControl/SimpleTorqueLimitingandGovernorController/RequestedTorqueSelection/MinMaxGovernorSelection ==
  BusTorqueLimit_Nm : Inport
  GovernorIndicatedTorqueFromGovernor : Inport  Port=2
  GovernorMode : Inport  Port=3
  GovernorTypeDefault : Inport  Port=4
  Compare To Constant : simulink/Logic and Bit Operations/Compare To Constant  relop=~=  const=-1  OutDataTypeStr=boolean
  MinMaxGovernorCommandLimiting_demand : MultiPortSwitch  DataPortOrder=Zero-based contiguous  zeroidx=on
  MinSpeedGovLimit : MinMax  Function=max  Inputs=2
  Switch : Switch  Criteria=u2 ~= 0
  zero limit2 : MinMax  Inputs=2
  GovernorIndicatedTorque : Outport
  wires:
  MinSpeedGovLimit/1 -> MinMaxGovernorCommandLimiting_demand/2
  Compare To Constant/1 -> zero limit2/1, MinSpeedGovLimit/2, MinMaxGovernorCommandLimiting_demand/3
  GovernorIndicatedTorqueFromGovernor/1 -> zero limit2/2, Switch/1, MinSpeedGovLimit/1
  MinMaxGovernorCommandLimiting_demand/1 -> Switch/3  "RequestedIndicatedTorqueBeforeLimitsMinMax"
  Switch/1 -> GovernorIndicatedTorque/1  "RequestedIndicatedTorqueBeforeLimits"
  BusTorqueLimit_Nm/1 -> Compare To Constant/1
  GovernorTypeDefault/1 -> Switch/2
  zero limit2/1 -> MinMaxGovernorCommandLimiting_demand/4
  GovernorMode/1 -> MinMaxGovernorCommandLimiting_demand/1

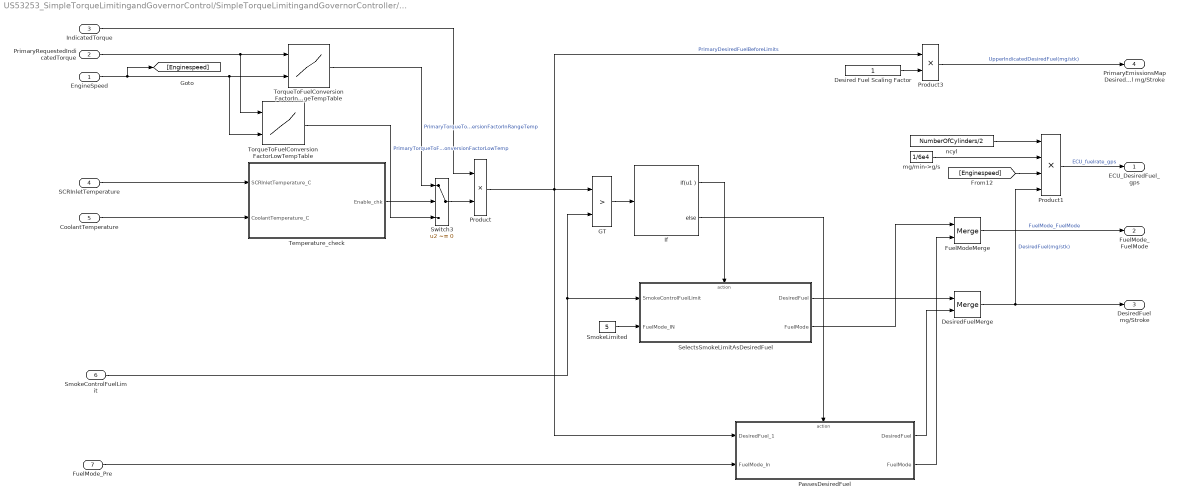
== system US53253_SimpleTorqueLimitingandGovernorControl/SimpleTorqueLimitingandGovernorController/Torque Based DesiredFuelDetermination(5ms)1/DesiredFuel ==
  EngineSpeed : Inport
  PrimaryRequestedIndicatedTorque : Inport  Port=2
  IndicatedTorque : Inport  Port=3
  SCRInletTemperature : Inport  Port=4
  CoolantTemperature : Inport  Port=5
  SmokeControlFuelLimit : Inport  Port=6
  FuelMode_Pre : Inport  Port=7
  Desired Fuel Scaling Factor : Constant
  DesiredFuelMerge : Merge
  FuelModeMerge : Merge
  GT : RelationalOperator  Operator=>  OutDataTypeStr=boolean  RndMeth=Nearest
  If : If  IfExpression=u1
  PassesDesiredFuel : Subsystem  TreatAsAtomicUnit=on
  Product : Product  RndMeth=Zero
  Product1 : Product  Inputs=****  RndMeth=Zero
  Product3 : Product  Inputs=**  RndMeth=Zero
  SelectsSmokeLimitAsDesiredFuel : Subsystem  TreatAsAtomicUnit=on
  SmokeLimited : Constant  Value=5
  Switch3 : Switch  Criteria=u2 ~= 0
  Temperature_check : Subsystem
  TorqueToFuelConversionFactorInRangeTempTable : Lookup_n-D  BreakpointsForDimension1=TorqueToFuelConversionFactorInRangeTempTable_Y  BreakpointsForDimension2=TorqueToFuelConversionFactorInRangeTable_X  Table=TorqueToFuelConversionFactorInRangeTempTable  ExtrapMethod=Clip  UseLastTableValue=on  RndMeth=Simplest  InputSameDT=on
  TorqueToFuelConversionFactorLowTempTable : Lookup_n-D  BreakpointsForDimension1=TorqueToFuelConversionFactorLowTempTable_Y  BreakpointsForDimension2=TorqueToFuelConversionFactorLowTempTable_X  Table=TorqueToFuelConversionFactorLowTempTable  ExtrapMethod=Clip  UseLastTableValue=on  RndMeth=Simplest  InputSameDT=on
  mg/min->g/s : Constant  Value=1/6e4
  ncyl : Constant  Value=NumberOfCylinders/2
  ECU_DesiredFuel_gps : Outport
  FuelMode_FuelMode : Outport  Port=2
  DesiredFuel mg/Stroke : Outport  Port=3
  PrimaryEmissionsMapDesiredFuel mg/Stroke : Outport  Port=4
  wires:
  IndicatedTorque/1 -> Product/1
  Product/1 -> Product3/1, PassesDesiredFuel/1(DesiredFuel_1), GT/1  "PrimaryDesiredFuelBeforeLimits"
  PrimaryRequestedIndicatedTorque/1 -> TorqueToFuelConversionFactorLowTempTable/1, TorqueToFuelConversionFactorInRangeTempTable/1
  TorqueToFuelConversionFactorLowTempTable/1 -> Switch3/3  "PrimaryTorqueToFuelConversionFactorLowTemp"
  TorqueToFuelConversionFactorInRangeTempTable/1 -> Switch3/1  "PrimaryTorqueToFuelConversionFactorInRangeTemp"
  CoolantTemperature/1 -> Temperature_check/2(CoolantTemperature_C)
  Temperature_check/1(Enable_chk) -> Switch3/2
  SCRInletTemperature/1 -> Temperature_check/1(SCRInletTemperature_C)
  Switch3/1 -> Product/2
  If/1 -> SelectsSmokeLimitAsDesiredFuel/Action
  DesiredFuelMerge/1 -> DesiredFuel mg/Stroke/1, Product1/4  "DesiredFuel(mg/stk)"
  GT/1 -> If/1
  If/2 -> PassesDesiredFuel/Action
  SelectsSmokeLimitAsDesiredFuel/1(DesiredFuel) -> DesiredFuelMerge/1
  PassesDesiredFuel/1(DesiredFuel) -> DesiredFuelMerge/2
  FuelModeMerge/1 -> FuelMode_FuelMode/1  "FuelMode_FuelMode"
  SmokeLimited/1 -> SelectsSmokeLimitAsDesiredFuel/2(FuelMode_IN)
  SelectsSmokeLimitAsDesiredFuel/2(FuelMode) -> FuelModeMerge/1
  PassesDesiredFuel/2(FuelMode) -> FuelModeMerge/2
  FuelMode_Pre/1 -> PassesDesiredFuel/2(FuelMode_In)
  SmokeControlFuelLimit/1 -> GT/2, SelectsSmokeLimitAsDesiredFuel/1(SmokeControlFuelLimit)
  Product1/1 -> ECU_DesiredFuel_gps/1  "ECU_fuelrate_gps"
  ncyl/1 -> Product1/1
  mg/min->g/s/1 -> Product1/2
  [Enginespeed] -> Product1/3
  Product3/1 -> PrimaryEmissionsMapDesiredFuel mg/Stroke/1  "UpperIndicatedDesiredFuel(mg/stk)"
  Desired Fuel Scaling Factor/1 -> Product3/2
  EngineSpeed/1 -> [Enginespeed], TorqueToFuelConversionFactorInRangeTempTable/2, TorqueToFuelConversionFactorLowTempTable/2

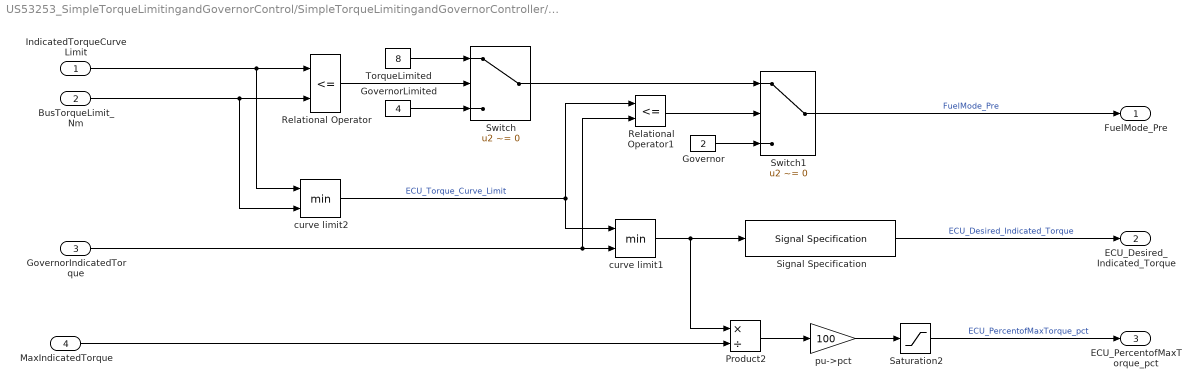
== system US53253_SimpleTorqueLimitingandGovernorControl/SimpleTorqueLimitingandGovernorController/Torque Based DesiredFuelDetermination(5ms)1/FuelModeAndTorqueConversionCalculaions ==
  IndicatedTorqueCurveLimit : Inport
  BusTorqueLimit_Nm : Inport  Port=2
  GovernorIndicatedTorque : Inport  Port=3
  MaxIndicatedTorque : Inport  Port=4
  Governor : Constant  Value=2
  GovernorLimited : Constant  Value=4
  Product2 : Product  Inputs=*/  RndMeth=Zero
  Relational Operator : RelationalOperator  Operator=<=  OutDataTypeStr=boolean  RndMeth=Nearest
  Relational Operator1 : RelationalOperator  Operator=<=  OutDataTypeStr=boolean  RndMeth=Nearest
  Saturation2 : Saturate  UpperLimit=125  LowerLimit=-125
      settings: AttributesFormatString=<lim: %<LowerLimit>/%<UpperLimit>>
  Signal Specification : SignalSpecification  Dimensions=1
  Switch : Switch  Criteria=u2 ~= 0
  Switch1 : Switch  Criteria=u2 ~= 0
  TorqueLimited : Constant  Value=8
  curve limit1 : MinMax  Inputs=2
  curve limit2 : MinMax  Inputs=2
  pu->pct : Gain  Gain=100
  FuelMode_Pre : Outport
  ECU_Desired_Indicated_Torque : Outport  Port=2
  ECU_PercentofMaxTorque_pct : Outport  Port=3
  wires:
  pu->pct/1 -> Saturation2/1
  Product2/1 -> pu->pct/1
  Saturation2/1 -> ECU_PercentofMaxTorque_pct/1  "ECU_PercentofMaxTorque_pct"
  curve limit1/1 -> Product2/1, Signal Specification/1
  IndicatedTorqueCurveLimit/1 -> Relational Operator/1, curve limit2/1
  GovernorIndicatedTorque/1 -> curve limit1/2, Relational Operator1/2
  MaxIndicatedTorque/1 -> Product2/2
  Signal Specification/1 -> ECU_Desired_Indicated_Torque/1  "ECU_Desired_Indicated_Torque"
  Relational Operator1/1 -> Switch1/2
  Switch1/1 -> FuelMode_Pre/1  "FuelMode_Pre"
  BusTorqueLimit_Nm/1 -> Relational Operator/2, curve limit2/2
  curve limit2/1 -> curve limit1/1, Relational Operator1/1  "ECU_Torque_Curve_Limit"
  Governor/1 -> Switch1/3
  Relational Operator/1 -> Switch/2
  TorqueLimited/1 -> Switch/1
  GovernorLimited/1 -> Switch/3
  Switch/1 -> Switch1/1
